simulink model "baro_block"  (R2025b)
settings: Solver=VariableStepAuto  StartTime=0.0  StopTime=10.0  RelTol=1e-3
values from neighbouring files (symbols this model uses):
  Baro = evalin('base', 'Baro')    [casper_baro_step.m]    (also in test_baro_model.m)
settings Model: Creator=Ashwin  LastModifiedBy=Ashwin

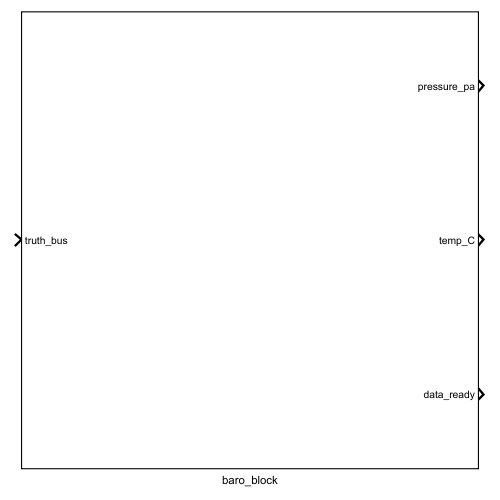
[thumbnail: Simulink's stored preview of the top-level diagram]
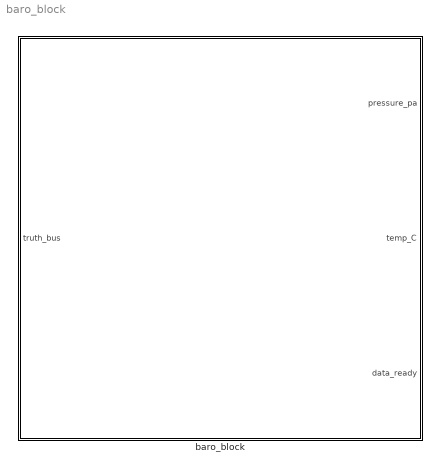
== system baro_block ==
  baro_block : Subsystem

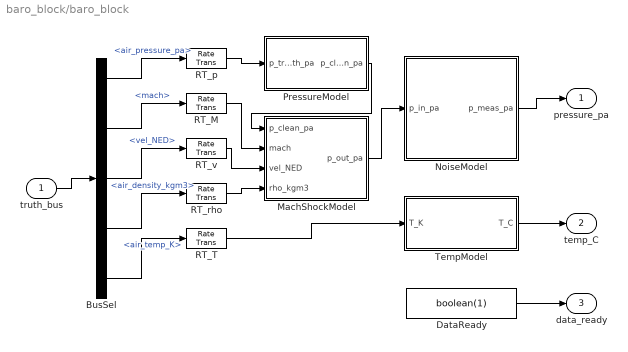
== system baro_block/baro_block ==
  truth_bus : Inport  OutDataTypeStr=Bus: TruthBus
  BusSel : BusSelector  OutputSignals=air_pressure_pa,mach,vel_NED,air_density_kgm3,air_temp_K
  DataReady : Constant  Value=boolean(1)  OutDataTypeStr=boolean  SampleTime=1/Baro.Rate_Hz
  MachShockModel : MATLAB Function  TreatAsAtomicUnit=on
  NoiseModel : MATLAB Function  TreatAsAtomicUnit=on
  PressureModel : MATLAB Function  TreatAsAtomicUnit=on
  RT_M : RateTransition  OutPortSampleTime=1/Baro.Rate_Hz
  RT_T : RateTransition  OutPortSampleTime=1/Baro.Rate_Hz
  RT_p : RateTransition  OutPortSampleTime=1/Baro.Rate_Hz
  RT_rho : RateTransition  OutPortSampleTime=1/Baro.Rate_Hz
  RT_v : RateTransition  OutPortSampleTime=1/Baro.Rate_Hz
  TempModel : MATLAB Function  TreatAsAtomicUnit=on
  pressure_pa : Outport
  temp_C : Outport  Port=2
  data_ready : Outport  Port=3
  wires:
  truth_bus/1 -> BusSel/1
  BusSel/1 -> RT_p/1  "<air_pressure_pa>"
  BusSel/2 -> RT_M/1  "<mach>"
  BusSel/3 -> RT_v/1  "<vel_NED>"
  BusSel/4 -> RT_rho/1  "<air_density_kgm3>"
  BusSel/5 -> RT_T/1  "<air_temp_K>"
  RT_p/1 -> PressureModel/1(p_truth_pa)
  PressureModel/1(p_clean_pa) -> MachShockModel/1(p_clean_pa)
  RT_M/1 -> MachShockModel/2(mach)
  RT_v/1 -> MachShockModel/3(vel_NED)
  RT_rho/1 -> MachShockModel/4(rho_kgm3)
  MachShockModel/1(p_out_pa) -> NoiseModel/1(p_in_pa)
  RT_T/1 -> TempModel/1(T_K)
  NoiseModel/1(p_meas_pa) -> pressure_pa/1
  TempModel/1(T_C) -> temp_C/1
  DataReady/1 -> data_ready/1

== matlab function baro_block/MachShockModel ==
  data: p_clean_pa input size=1; p_out_pa output size=1; mach input size=1; vel_NED input size=[3 1]; rho_kgm3 input size=1
function p_out_pa = fcn(p_clean_pa, mach, vel_NED, rho_kgm3)
%#codegen
p_out_pa = casper_baro_mach_shock(p_clean_pa, mach, vel_NED, rho_kgm3);
end

== matlab function baro_block/PressureModel ==
  data: p_truth_pa input size=1; p_clean_pa output size=1
function p_clean_pa = fcn(p_truth_pa)
%#codegen
p_clean_pa = casper_baro_pressure_model(p_truth_pa);
end

== matlab function baro_block/NoiseModel ==
  data: p_in_pa input size=1; p_meas_pa output size=1
function p_meas_pa = fcn(p_in_pa)
%#codegen
p_meas_pa = double(0);
coder.extrinsic('casper_baro_noise_step');
p_meas_pa = casper_baro_noise_step(p_in_pa);
end

== matlab function baro_block/TempModel ==
  data: T_K input size=1; T_C output size=1
function T_C = fcn(T_K)
%#codegen
T_C = T_K - 273.15;
end
